simulink model "LAFES"  (R2024a)
settings: Solver=FixedStepAuto  StartTime=0.0  StopTime=3600  FixedStep=0.01  RelTol=1e-3
PreLoadFcn:
  | addpath(genpath('./S_Functions'))
InitFcn:
  | NETIF =  'eth0';
model workspace (MAT data in the model file):
  Sig = Simulink.Signal
  Sig.DataType = 'auto'
  Sig.Dimensions = -1
  Sig.DimensionsMode = 'auto'
  Sig.Complexity = 'auto'
  Sig.SampleTime = -1
  Sig.SamplingMode = 'auto'
  link_id = 1
  main_switch = Simulink.Parameter
  main_switch.Value = 1
  main_switch.Complexity = 'real'
  main_switch.Dimensions = [1 1]
  main_switch.DataType = 'boolean'
  quick_stop = Simulink.Parameter
  quick_stop.Value = 0
  quick_stop.Complexity = 'real'
  quick_stop.Dimensions = [1 1]
  quick_stop.DataType = 'boolean'
  useGenerator = Simulink.Parameter
  useGenerator.Value = 1
  useGenerator.Complexity = 'real'
  useGenerator.Dimensions = [1 1]
  useGenerator.DataType = 'boolean'
settings Model: SimulationMode=external  Creator=20192648  LastModifiedBy=20201350
settings HardwareCC: ProdBitPerLong=64  ProdHWDeviceType=Intel->x86-64 (Linux 64)
settings ModelReferenceCC: EnableRefExpFcnMdlSchedulingChecks=on  PropagateSignalLabelsOutOfModel=off
settings RTWCC: Description=RoboCup Realtime Target  SystemTargetFile=mttarget.tlc  MakeCommand="make_rtw CC=\"ccache gcc\" OPTS=\"-DNETIF_ID=0 -DTEST_CONN_MODEL -D_GNU_SOURCE -DPRIO=99\""  TemplateMakefile=mt_unix.tmf  CustomInclude=./S_Functions  RTWCompilerOptimization=Custom  RTWCustomCompilerOptimizations=-O2 -g -W
settings RTWCC: CustomSource=|
  | Rs485EthercatLibrary.c
  | ethercatbase.c
  | ethercatcoe.c
  | ethercatconfig.c
  | ethercatdc.c
  | ethercatfoe.c
  | ethercatmain.c
  | ethercatprint.c
  | ethercatsoe.c
  | nicdrv.c
  | osal.c
  | oshw.c
  | timer_posix.c
  | timer_stats.c
settings CodeAppCC: StateflowObjectComments=on
settings GRTTargetCC: TargetLangStandard=C89/C90 (ANSI)  CodeReplacementLibrary=GNU C99 extensions  UseToolchainInfoCompliant=off  ExtMode=on

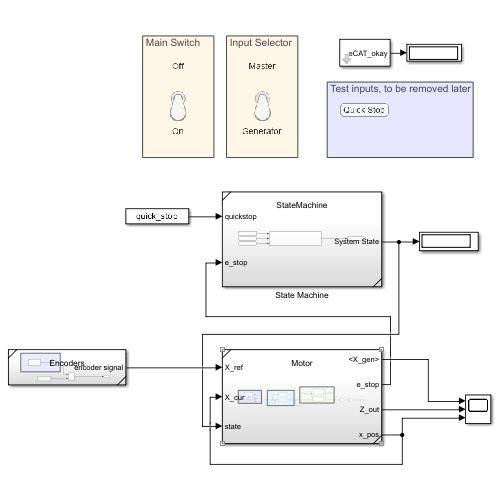
[thumbnail: Simulink's stored preview of the top-level diagram]
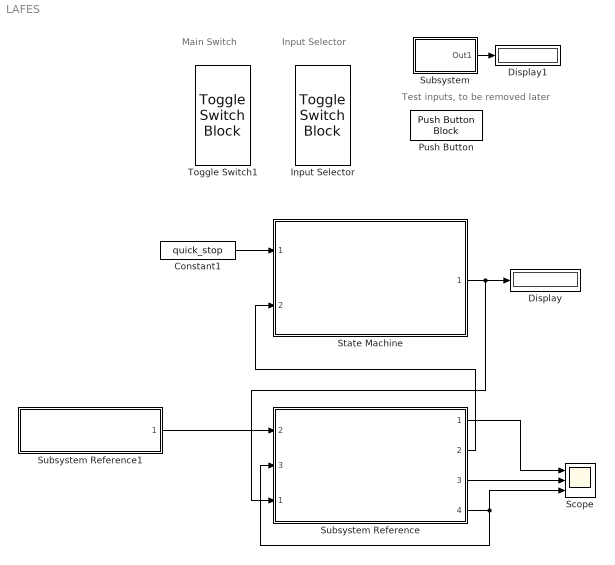
== system LAFES ==
  note: Test inputs, to be removed later
  note: Input Selector
  note: Main Switch
  Constant1 : Constant  Value=quick_stop
  Display : Display
  Display1 : Display
  Input Selector : ToggleSwitchBlock  LabelPosition=Hide
      settings: Values={{'Generator', 'Master'}, [1 0]}
  Push Button : PushButtonBlock  ButtonText=Quick Stop  ButtonType=Latch
  Scope : Scope  NumInputPorts=3
  State Machine : Subsystem  ReferencedSubsystem=StateMachine
  Subsystem : Subsystem  mask{NETIF=NETIF}
  Subsystem Reference : Subsystem  ReferencedSubsystem=Motor
      settings: PortSchema="{\"entries\":[{\"content\":{\"sides\":[{\"content\":{\"connectorIds\":[\"In2\",\"In3\",\"In1\"]},\"type\":\"ConnectorPlacement.EquallySpacedRectSide\",\"uuid\":\"5e979ca3-cd75-44e9-8447-42d64532c21d\"},{\"content\":{\"connectorIds\":[\"Out1\",\"Out2\",\"Out3\",\"Out4\"],\"side\":\"RIGHT\"},\"type\":\"ConnectorPlacement.EquallySpacedRectSide\",\"uuid\":\"fc5069ac-6226-4adb-b296-a272106e9449\"},{\"content\":{\"side\":\"TOP\"},\"type\":\"ConnectorPlacement.EquallySpacedRectSide\",\"uuid\":\"3eaed910-23b4-461f-88ca-88f61c390ce5\"}]},\"type\":\"ConnectorPlacement.EquallySpacedConnector\",\"uuid\":\"b260754b-f789-4d67-9165-cc44557c7df2\"}],\"packageUris\":[\"http://schema.mathworks.com/mf0/Connector/R2020b\"],\"version\":\"1.0\"}"
  Subsystem Reference1 : Subsystem  ReferencedSubsystem=Encoders
  Toggle Switch1 : ToggleSwitchBlock  LabelPosition=Hide
      settings: Values={{'On', 'Off'}, [1 0]}
  wires:
  Subsystem/1(Out1) -> Display1/1
  Constant1/1 -> State Machine/1
  Subsystem Reference/2 -> State Machine/2
  State Machine/1 -> Subsystem Reference/1, Display/1
  Subsystem Reference/4 -> Subsystem Reference/3, Scope/3
  Subsystem Reference/3 -> Scope/2
  Subsystem Reference/1 -> Scope/1
  Subsystem Reference1/1 -> Subsystem Reference/2

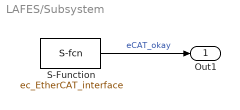
== system LAFES/Subsystem ==
  S-Function : S-Function  FunctionName=ec_EtherCAT_interface  Parameters=NETIF  SFunctionDeploymentMode=off  EnableBusSupport=off
  Out1 : Outport
  wires:
  S-Function/1 -> Out1/1  "eCAT_okay"
